simulink library "INT_Tra_Prt"  (R2016b)
settings: Solver=VariableStepAuto  StartTime=0.0  StopTime=10.0  RelTol=1e-3
settings Model: Creator=Administrator  LastModifiedBy=Administrator

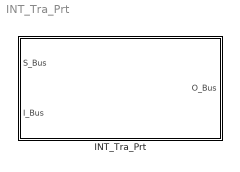
== system INT_Tra_Prt ==
  INT_Tra_Prt : Subsystem

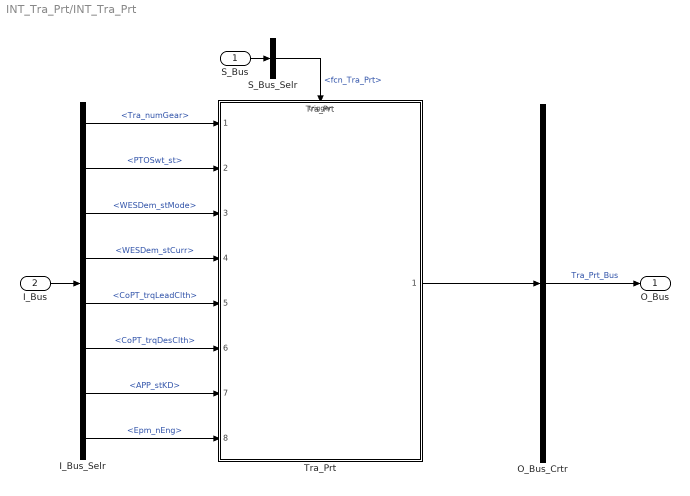
== system INT_Tra_Prt/INT_Tra_Prt ==
  S_Bus : Inport
  I_Bus : Inport  Port=2
  I_Bus_Selr : BusSelector  OutputSignals=Tra_numGear,PTOSwt_st,WESDem_stMode,WESDem_stCurr,CoPT_trqLeadClth,CoPT_trqDesClth,APP_stKD,Epm_nEng
  O_Bus_Crtr : BusCreator  Inputs=1
  S_Bus_Selr : BusSelector  OutputSignals=fcn_Tra_Prt
  Tra_Prt : ModelReference  ModelNameDialog=Tra_Prt  SimulationMode=Normal  ModelReferenceVersion=1.22  TriggerPortName=function  TriggerPortTriggerType=function-call  TriggerPortStatesWhenEnabling=held
  O_Bus : Outport
  wires:
  S_Bus_Selr/1 -> Tra_Prt/Trigger  "<fcn_Tra_Prt>"
  S_Bus/1 -> S_Bus_Selr/1
  I_Bus/1 -> I_Bus_Selr/1
  I_Bus_Selr/1 -> Tra_Prt/1  "<Tra_numGear>"
  I_Bus_Selr/2 -> Tra_Prt/2  "<PTOSwt_st>"
  I_Bus_Selr/3 -> Tra_Prt/3  "<WESDem_stMode>"
  I_Bus_Selr/4 -> Tra_Prt/4  "<WESDem_stCurr>"
  I_Bus_Selr/5 -> Tra_Prt/5  "<CoPT_trqLeadClth>"
  I_Bus_Selr/6 -> Tra_Prt/6  "<CoPT_trqDesClth>"
  I_Bus_Selr/7 -> Tra_Prt/7  "<APP_stKD>"
  I_Bus_Selr/8 -> Tra_Prt/8  "<Epm_nEng>"
  O_Bus_Crtr/1 -> O_Bus/1  "Tra_Prt_Bus"
  Tra_Prt/1 -> O_Bus_Crtr/1
